simulink model "slosh_attitude_sim"  (R2025a)
settings: Solver=ode45  StartTime=0.0  StopTime=80  MaxStep=0.01  RelTol=1e-6
settings Model: Creator=alexsolakhyan  LastModifiedBy=alexsolakhyan
settings DataIOCC: SaveState=on

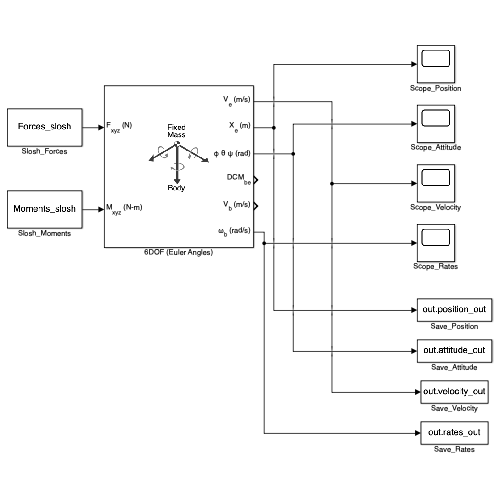
[thumbnail: Simulink's stored preview of the top-level diagram]
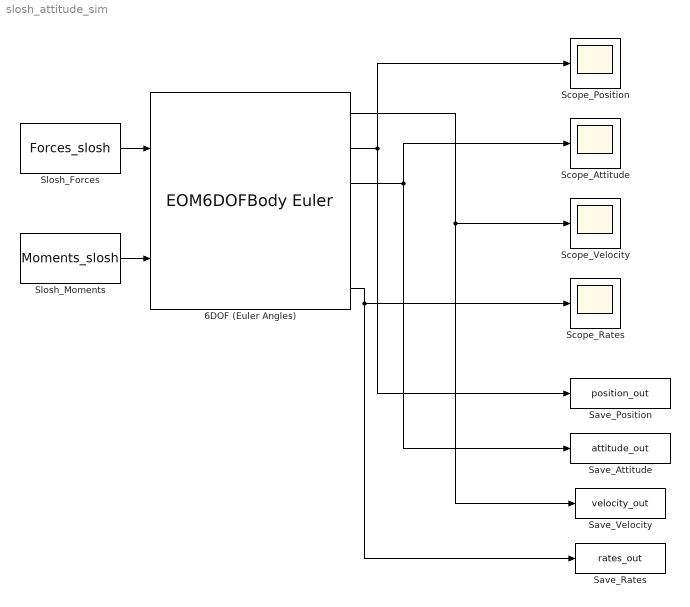
== system slosh_attitude_sim ==
  6DOF (Euler Angles) : EOM6DOFBodyEuler  mass_0=205.112  inertia=[ 36.25 0 0; 0 29.7478 0; 0 0 44.8639]
  Save_Attitude : ToWorkspace  VariableName=attitude_out  SaveFormat=Structure With Time  SampleTime=-1
  Save_Position : ToWorkspace  VariableName=position_out  SaveFormat=Structure With Time  SampleTime=-1
  Save_Rates : ToWorkspace  VariableName=rates_out  SaveFormat=Structure With Time  SampleTime=-1
  Save_Velocity : ToWorkspace  VariableName=velocity_out  SaveFormat=Structure With Time  SampleTime=-1
  Scope_Attitude : Scope
      settings: ActiveDisplayYMinimum=-3.9458057371502488  ActiveDisplayYMaximum=4.5491531936608345  DataLoggingVariableName=Scope_Attitude
  Scope_Position : Scope
      settings: ActiveDisplayYMinimum=-0.1326789750311145  ActiveDisplayYMaximum=0.052336715436328209  DataLoggingVariableName=Scope_Position
  Scope_Rates : Scope
      settings: ActiveDisplayYMinimum=-0.090707233355600353  ActiveDisplayYMaximum=0.036777931104880444  DataLoggingVariableName=Scope_Rates
  Scope_Velocity : Scope
      settings: ActiveDisplayYMinimum=-0.0013404113962990089  ActiveDisplayYMaximum=0.000875627219524438  DataLoggingVariableName=Scope_Velocity
  Slosh_Forces : FromWorkspace  VariableName=Forces_slosh  OutputAfterFinalValue=Setting to zero
  Slosh_Moments : FromWorkspace  VariableName=Moments_slosh  OutputAfterFinalValue=Setting to zero
  wires:
  Slosh_Forces/1 -> 6DOF (Euler Angles)/1
  Slosh_Moments/1 -> 6DOF (Euler Angles)/2
  6DOF (Euler Angles)/1 -> Save_Velocity/1, Scope_Velocity/1
  6DOF (Euler Angles)/3 -> Save_Attitude/1, Scope_Attitude/1
  6DOF (Euler Angles)/2 -> Scope_Position/1, Save_Position/1
  6DOF (Euler Angles)/6 -> Scope_Rates/1, Save_Rates/1
